simulink model "ballast_node"  (Simulink 7.8)
settings: Solver=FixedStepDiscrete  SolverMode=SingleTasking  StartTime=0.0  StopTime=10.0  FixedStep=0.01  RelTol=1e-3
InitFcn:
  | clear all
  | common
  | BallastBusses
undefined symbols (not defined in the file or in its folder): ANmax, BallastEcanInit, BallastNodeInit, Init_onlyOnce, Init_Reset, SendAndReceiveEcan, T_step
libraries: dsPICdrivers x11, simulink x6
settings Model: Creator=bwmairs  LastModifiedBy=Bryant
settings OptimizationCC: InlineParams=on  InlineInvariantSignals=on  InitFltsAndDblsToZero=on  EfficientFloat2IntCast=on
settings DebuggingCC: ReadBeforeWriteMsg=DisableAll  WriteAfterWriteMsg=DisableAll  WriteAfterReadMsg=DisableAll  UnderspecifiedInitializationDetection=Simplified  ParameterOverflowMsg=warning  FcnCallInpInsideContextMsg=Use local settings  UniqueDataStoreMsg=error
settings HardwareCC: ProdBitPerInt=16  ProdBitPerPointer=16  ProdIntDivRoundTo=Zero  ProdEndianess=LittleEndian  ProdWordSize=16  ProdHWDeviceType=16-bit Generic
settings ModelReferenceCC: ModelReferenceNumInstancesAllowed=Single
settings SFSimCC: SimParseCustomCode=off
settings RTWCC: SystemTargetFile=dspic.tlc  GenCodeOnly=on  MakeCommand=make_CreateMPLAB  TemplateMakefile=dspic_pic30_gcc.tmf  PostCodeGenCommand=dsPIC_Compile()  Description=Embedded Target for Microchip dsPIC (real-time)  ProcessScript=dspic_make_rtw_hook  RTWCompilerOptimization=On
settings RTWCC: CustomInclude=|
  | clib
  | ../Libs/C
settings RTWCC: CustomSource=|
  | clib/BallastNode.c
  | 
  | ../Libs/C/Node.c
  | ../Libs/C/Nmea2000.c
  | ../Libs/C/Nmea2000Encode.c
  | ../Libs/C/DEE.c
  | ../Libs/C/DEES_33F_24F.s
  | ../Libs/C/MessageScheduler.c
  | ../Libs/C/CanMessages.c
  | ../Libs/C/CircularBuffer.c
  | ../Libs/C/Ecan1.c
  | ../Libs/C/Parameters.c
  | ../Libs/C/ParametersHelper.c
  | ../Libs/C/DataStore.c
settings STFCustomTargetCC: TargetFunctionLibrary=C89/C90 (ANSI)  IncludeMdlTerminateFcn=off  SupportNonInlinedSFcns=off  SystemTargetFile=dspic.tlc
settings ERTTargetCC: TargetFunctionLibrary=C89/C90 (ANSI)  MultiwordLength=2048  ParMdlRefBuildCompliant=off  CompOptLevelCompliant=off  ConcurrentExecutionCompliant=off  IncludeMdlTerminateFcn=off  GeneratePreprocessorConditionals=Disable all  CombineOutputUpdateFcns=off  ERTFirstTimeCompliant=off  ERTCustomFileBanners=off  SupportContinuousTime=on  ModelStepFunctionPrototypeControlCompliant=off  CPPClassGenCompliant=off  ExtModeMexFile=ext_serial_win32_comm  InlinedParameterPlacement=NonHierarchical  ERTSrcFileBannerTemplate=dsPIC_code_template.cgt  ERTHdrFileBannerTemplate=dsPIC_code_template.cgt  ERTDataSrcFileTemplate=dsPIC_code_template.cgt  ERTDataHdrFileTemplate=dsPIC_code_template.cgt  ERTCustomFileTemplate=dsPIC_main.tlc  ConvertIfToSwitch=off  SuppressUnreachableDefaultCases=off
settings CustomProperty: DataType=string  Value=C:\PROGRA~1\MATLAB\R2011b\bin\win64\gmake

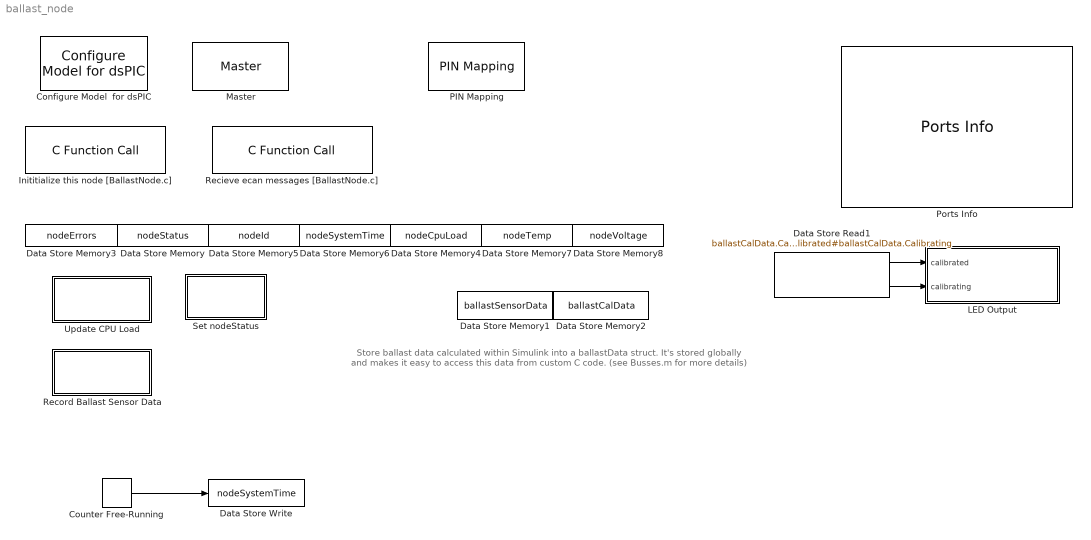
== system ballast_node ==
  note: Store ballast data calculated within Simulink into a ballastData struct.
      | It's stored globally and makes it easy to access this data from custom
      | C code. (see Busses.m for more details)
  Configure Model  for dsPIC : dsPICdrivers/Simulink Configuration/Configure Model  for dsPIC
  Counter Free-Running : simulink/Sources/Counter Free-Running  NumBits=32  tsamp=T_step
  Data Store Memory : DataStoreMemory  DataStoreName=nodeStatus  ReadBeforeWriteMsg=warning  WriteAfterWriteMsg=warning  WriteAfterReadMsg=warning  OutDataTypeStr=uint16
      settings: RTWStateStorageClass=ImportedExtern
  Data Store Memory1 : DataStoreMemory  DataStoreName=ballastSensorData  ReadBeforeWriteMsg=warning  WriteAfterWriteMsg=warning  WriteAfterReadMsg=warning  OutDataTypeStr=Bus: BallastVariables
      settings: RTWStateStorageClass=ImportedExtern
  Data Store Memory2 : DataStoreMemory  DataStoreName=ballastCalData  ReadBeforeWriteMsg=warning  WriteAfterWriteMsg=warning  WriteAfterReadMsg=warning  OutDataTypeStr=Bus: BallastCalData
      settings: RTWStateStorageClass=ImportedExtern
  Data Store Memory3 : DataStoreMemory  DataStoreName=nodeErrors  ReadBeforeWriteMsg=warning  WriteAfterWriteMsg=warning  WriteAfterReadMsg=warning  OutDataTypeStr=uint16
      settings: RTWStateStorageClass=ImportedExtern
  Data Store Memory4 : DataStoreMemory  DataStoreName=nodeCpuLoad  ReadBeforeWriteMsg=warning  WriteAfterWriteMsg=warning  WriteAfterReadMsg=warning  OutDataTypeStr=uint8
      settings: RTWStateStorageClass=ImportedExtern
  Data Store Memory5 : DataStoreMemory  DataStoreName=nodeId  ReadBeforeWriteMsg=warning  WriteAfterWriteMsg=warning  WriteAfterReadMsg=warning  OutDataTypeStr=uint8
      settings: RTWStateStorageClass=ImportedExtern
  Data Store Memory6 : DataStoreMemory  DataStoreName=nodeSystemTime  ReadBeforeWriteMsg=warning  WriteAfterWriteMsg=warning  WriteAfterReadMsg=warning  OutDataTypeStr=uint32
      settings: RTWStateStorageClass=ImportedExtern
  Data Store Memory7 : DataStoreMemory  DataStoreName=nodeTemp  ReadBeforeWriteMsg=warning  WriteAfterWriteMsg=warning  WriteAfterReadMsg=warning  OutDataTypeStr=int8
      settings: RTWStateStorageClass=ImportedExtern
  Data Store Memory8 : DataStoreMemory  DataStoreName=nodeVoltage  ReadBeforeWriteMsg=warning  WriteAfterWriteMsg=warning  WriteAfterReadMsg=warning  OutDataTypeStr=uint8
      settings: RTWStateStorageClass=ImportedExtern
  Data Store Read1 : DataStoreRead  DataStoreName=ballastCalData  SampleTime=T_step  DataStoreElements=ballastCalData.Calibrated#ballastCalData.Calibrating
  Data Store Write : DataStoreWrite  DataStoreName=nodeSystemTime
  Inititialize this node [BallastNode.c] : dsPICdrivers/OTHERS/C Function Call  Tag=dsPIC_dsPIC_CFunctionCall  FctUpdate=None  fctName=BallastEcanInit  INPUT_SIZE=1  INPUT1=--  INPUT2=--  INPUT3=--  OUTPUT_SIZE=-1  OUTPUT1=--  SampleTime=Inf  InputType=[]  OutputType=[]  FctDeclaration=extern void BallastEcanInit();  FctCall=BallastEcanInit();  OrderingInOutPopup=None  FctStart=Start Function (Call once and only once)  FctStart_Name=BallastNodeInit  FctStart_Declaration=inline extern void BallastNodeInit();  FctStart_Call=BallastNodeInit();  FctInit=None  FctInit_Name=BallastEcanInit  FctInit_Declaration=inline extern void BallastEcanInit();  FctInit_Call=BallastEcanInit();  PinDigitalInput=[]  PinDigitalOutput=[]  AnalogueInput=[]
  LED Output : Subsystem
  Master : dsPICdrivers/Master  Tag=dsPIC_MASTER  Priority=1  TimeStepType=Timer1  picType=33fj128MC802  fcy=40008571.4286  Quartz_33f=8e6  PLLActive_33f=on  fcyDesired_33f=40000000  tmr1="[8  50010  -0.00057131]"  tmr1Info="Time Step : 0.01  ;   Error : -0.00057131%  PR1=50010"  tmr2345="[0  0  0  0]"  tmr2345cfg=[-1 -1 -1 -1]  IOautoConf=on  typePort="[ 9   8   0   0  10   0   0   0   0   0   0   0   0   0   0   0   0   9   8   8  22   0   0  23   0   0   0   0  23   0   0   0   0   0   0   0   0   0   0   0   0   0   0   0   0   0   0   0   0   0   0   0   0   0   0   0   0   0   0   0   0   0   0   0   0   0   0   0   0   0   0   0   0   0   0   0   0   0   0   0   0   0   0   0   0   0   0   0   0   0   0   0   0   0   0   0   0   0   0   0   0   0   0   0   0   0   0   0   0   0   0   0 ]"  TRIS="[ 65519  61311  65535  65535  65535  65535  65535 ]"  ADPCFG=9  MasterBusyPort=None  MasterOverloadPort=None  FOSC=Internal Fast RC 7.37Mhz  ClockSwitchMonitor=Both disabled  TempProtection_33f=TEMP_ON  FPBOR=<empty>  PWRT=disable  MCLR=<empty>  ICD=ICS_PGD3  JTAGEN=JTAGEN_OFF  PowerSave=off  OverrideFcy=off  NewFcy=1e6  PR2345="[65535  65535  65535  65535]"
  PIN Mapping : dsPICdrivers/Peripheral MAPPING/PIN Mapping  Tag=dsPIC_PIN_Mapping  in_INT1=Not tied (VSS)  in_INT2=Not tied (VSS)  in_T2CK=Not tied (VSS)  in_T3CK=Not tied (VSS)  in_T4CK=Not tied (VSS)  in_T5CK=Not tied (VSS)  in_IC1=Not tied (VSS)  in_IC2=Not tied (VSS)  in_IC7=Not tied (VSS)  in_IC8=Not tied (VSS)  out_OC1=tied to RP12  out_OC2=Not changed  out_OC3=Not changed  out_OC4=Not changed  in_OCFA=Not tied (VSS)  in_FLTA1=Not tied (VSS)  in_FLTA2=Not tied (VSS)  in_QEA1=Not tied (VSS)  in_QEB1=Not tied (VSS)  in_INDX1=Not tied (VSS)  out_UPDN1=Not changed  out_UPDN2=Not changed  in_QEA2=Not tied (VSS)  in_QEB2=Not tied (VSS)  in_INDX2=Not tied (VSS)  in_U1RX=Not tied (VSS)  out_U1TX=Not changed  in_U1CTS=Not tied (VSS)  out_U1RTS=Not changed  in_U2RX=Not tied (VSS)  out_U2TX=Not changed  in_U2CTS=Not tied (VSS)  out_U2RTS=Not changed  in_SDI1=Not tied (VSS)  out_SDO1=Not changed  in_SCK1=Not tied (VSS)  out_SCK1OUT=Not changed  in_SS1=Not tied (VSS)  out_SS1OUT=Not changed  in_SDI2=Not tied (VSS)  out_SDO2=Not changed  in_SCK2=Not tied (VSS)  out_SCK2OUT=Not changed  in_SS2=Not tied (VSS)  out_SS2OUT=Not changed  in_C1RX=tied to RP4  out_C1TX=tied to RP7  out_C1OUT=Not changed  out_C2OUT=Not changed
  Ports Info : dsPICdrivers/Ports Info  Tag=dsPIC_PortInfo
  Recieve ecan messages [BallastNode.c] : dsPICdrivers/OTHERS/C Function Call  Tag=dsPIC_dsPIC_CFunctionCall  FctUpdate=Output Function  fctName=SendAndReceiveEcan  INPUT_SIZE=1  INPUT1=--  INPUT2=--  INPUT3=--  OUTPUT_SIZE=1  OUTPUT1=--  SampleTime=.01  InputType=[ ]  OutputType=[ ]  FctDeclaration=extern void SendAndReceiveEcan();  FctCall=SendAndReceiveEcan();  OrderingInOutPopup=None  FctStart=None  FctStart_Name=Init_onlyOnce  FctStart_Declaration=inline extern void Init_onlyOnce();  FctStart_Call=Init_onlyOnce();  FctInit=None  FctInit_Name=Init_Reset  FctInit_Declaration=inline extern void Init_Reset();  FctInit_Call=Init_Reset();  PinDigitalInput=[]  PinDigitalOutput=[]  AnalogueInput=[]
  Record Ballast Sensor Data : Subsystem
  Set nodeStatus : Subsystem
  Update CPU Load : Subsystem
      mask Display: disp('');
  wires:
  Data Store Read1/1 -> LED Output/1(calibrated)
  Data Store Read1/2 -> LED Output/2(calibrating)
  Counter Free-Running/1 -> Data Store Write/1

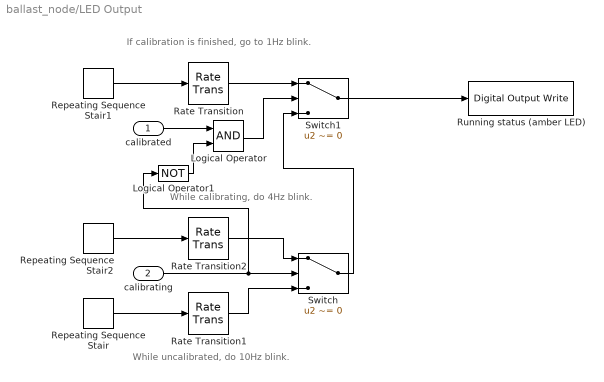
== system ballast_node/LED Output ==
  note: If calibration is finished, go to 1Hz blink.
  note: While calibrating, do 4Hz blink.
  note: While uncalibrated, do 10Hz blink.
  calibrated : Inport
  calibrating : Inport  Port=2
  Logical Operator : Logic  AllPortsSameDT=off  OutDataTypeStr=boolean
  Logical Operator1 : Logic  Operator=NOT  AllPortsSameDT=off  OutDataTypeStr=boolean
  Rate Transition : RateTransition
  Rate Transition1 : RateTransition
  Rate Transition2 : RateTransition
  Repeating Sequence Stair : simulink/Sources/Repeating Sequence Stair  OutValues=[1 0]  tsamp=.1  OutMin=[]  OutMax=[]  OutDataTypeStr=fixdt('boolean')  OutputDataTypeScalingMode=Specify via dialog  OutDataType=fixdt('boolean')  ConRadixGroup=Best Precision: Vector-wise  OutScaling=[]
  Repeating Sequence Stair1 : simulink/Sources/Repeating Sequence Stair  OutValues=[1 0]  tsamp=1  OutMin=[]  OutMax=[]  OutDataTypeStr=fixdt('boolean')  OutputDataTypeScalingMode=Specify via dialog  OutDataType=fixdt('boolean')  ConRadixGroup=Best Precision: Vector-wise  OutScaling=[]
  Repeating Sequence Stair2 : simulink/Sources/Repeating Sequence Stair  OutValues=[1 0]  tsamp=.25  OutMin=[]  OutMax=[]  OutDataTypeStr=fixdt('boolean')  OutputDataTypeScalingMode=Specify via dialog  OutDataType=fixdt('boolean')  ConRadixGroup=Best Precision: Vector-wise  OutScaling=[]
  Running status (amber LED) : dsPICdrivers/Digital I//O/Digital Output Write  Tag=dsPIC_Digital_Output  Priority=5  PORT=A  Pin=[4]  Simultaneous=off  OrderingInOutPopup=None
  Switch : Switch  Criteria=u2 ~= 0
  Switch1 : Switch  Criteria=u2 ~= 0
  wires:
  Repeating Sequence Stair/1 -> Rate Transition1/1
  Rate Transition1/1 -> Switch/3
  calibrating/1 -> Switch/2, Logical Operator1/1
  Repeating Sequence Stair1/1 -> Rate Transition/1
  Rate Transition/1 -> Switch1/1
  Repeating Sequence Stair2/1 -> Rate Transition2/1
  Rate Transition2/1 -> Switch/1
  Switch1/1 -> Running status (amber LED)/1
  Switch/1 -> Switch1/3
  calibrated/1 -> Logical Operator/1
  Logical Operator/1 -> Switch1/2
  Logical Operator1/1 -> Logical Operator/2

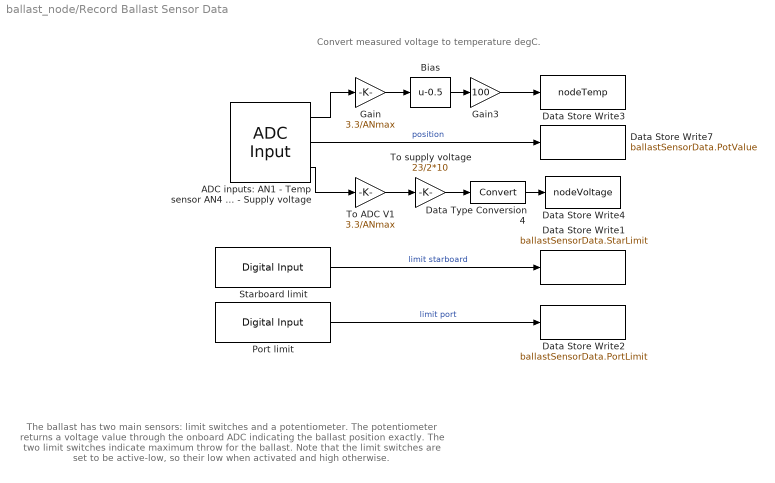
== system ballast_node/Record Ballast Sensor Data ==
  note: The ballast has two main sensors: limit switches and a potentiometer. The
      | potentiometer returns a voltage value through the onboard ADC indicating
      | the ballast position exactly. The two limit switches indicate maximum throw
      | for the ballast.
      |
      | Note that the limit switches are set to be active-low, so their low when activated
      | and high otherwise.
  note: Convert measured voltage to temperature degC.
  ADC inputs: AN1 - Temp sensor AN4 - Ballast pot AN5 - Supply voltage : dsPICdrivers/Peripheral I//O/ADC Input  Tag=dsPIC_ADC  Priority=5  ADC_TYPE=12 bits  ADC_MODE=Continuous sampling & get last channel value  NbrSampleStep=1  VoltRefpopup="AVdd  -  AVss"  OutFormatBitspopup=0000 dddd dddd dddd : Integer  InterruptPriority=6  ANCHANNELS=[4 5 1]  MaxName=ANmax = 4095  Rin=0  ADCS=53  SAMC=1  Temperature=25  DMAChannel=1  SampleTime=T_step  Status="OK  |  Tsmp=6.749e-007 |  T/Channel=1.012e-005 |  Tall=3.037e-005"  SSRC=auto convert
  Bias : Bias  Bias=-0.5
  Data Store Write1 : DataStoreWrite  DataStoreName=ballastSensorData  DataStoreElements=ballastSensorData.StarLimit
  Data Store Write2 : DataStoreWrite  DataStoreName=ballastSensorData  DataStoreElements=ballastSensorData.PortLimit
  Data Store Write3 : DataStoreWrite  DataStoreName=nodeTemp
  Data Store Write4 : DataStoreWrite  DataStoreName=nodeVoltage
  Data Store Write7 : DataStoreWrite  DataStoreName=ballastSensorData  DataStoreElements=ballastSensorData.PotValue
  Data Type Conversion4 : DataTypeConversion  RndMeth=Simplest
  Gain : Gain  Gain=3.3/ANmax  ParamDataTypeStr=single  OutDataTypeStr=single  RndMeth=Simplest
  Gain3 : Gain  Gain=100  ParamDataTypeStr=single  OutDataTypeStr=int8  RndMeth=Simplest
  Port limit : dsPICdrivers/Digital I//O/Digital Input  Tag=dsPIC_Digital_Input  PORT=A  Pin=[0]  SampleTime=T_step  OrderingInOutPopup=None
  Starboard limit : dsPICdrivers/Digital I//O/Digital Input  Tag=dsPIC_Digital_Input  PORT=B  Pin=[1]  SampleTime=T_step  OrderingInOutPopup=None
  To ADC V1 : Gain  Gain=3.3/ANmax
  To supply voltage : Gain  Gain=23/2*10  RndMeth=Simplest
  wires:
  Port limit/1 -> Data Store Write2/1  "limit port"
  Starboard limit/1 -> Data Store Write1/1  "limit starboard"
  ADC inputs: AN1 - Temp sensor AN4 - Ballast pot AN5 - Supply voltage/1 -> Gain/1
  Gain/1 -> Bias/1
  Bias/1 -> Gain3/1
  Gain3/1 -> Data Store Write3/1
  To ADC V1/1 -> To supply voltage/1
  ADC inputs: AN1 - Temp sensor AN4 - Ballast pot AN5 - Supply voltage/3 -> To ADC V1/1
  To supply voltage/1 -> Data Type Conversion4/1
  Data Type Conversion4/1 -> Data Store Write4/1
  ADC inputs: AN1 - Temp sensor AN4 - Ballast pot AN5 - Supply voltage/2 -> Data Store Write7/1  "position"

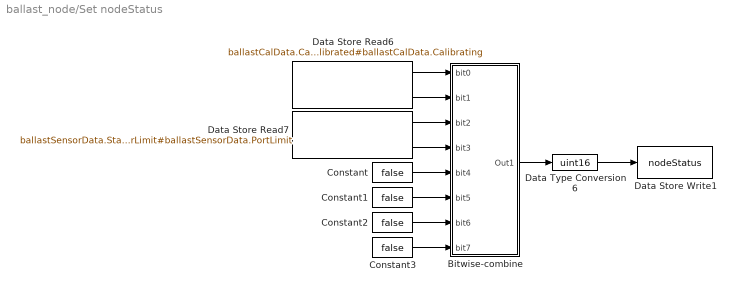
== system ballast_node/Set nodeStatus ==
  Bitwise-combine : Subsystem
  Constant{,1..3} (4 alike) : Constant  Value=false  OutDataTypeStr=boolean
  Data Store Read6 : DataStoreRead  DataStoreName=ballastCalData  SampleTime=T_step  DataStoreElements=ballastCalData.Calibrated#ballastCalData.Calibrating
  Data Store Read7 : DataStoreRead  DataStoreName=ballastSensorData  SampleTime=T_step  DataStoreElements=ballastSensorData.StarLimit#ballastSensorData.PortLimit
  Data Store Write1 : DataStoreWrite  DataStoreName=nodeStatus
  Data Type Conversion6 : DataTypeConversion  OutDataTypeStr=uint16
  wires:
  Constant/1 -> Bitwise-combine/5(bit4)
  Constant1/1 -> Bitwise-combine/6(bit5)
  Constant2/1 -> Bitwise-combine/7(bit6)
  Constant3/1 -> Bitwise-combine/8(bit7)
  Data Store Read6/1 -> Bitwise-combine/1(bit0)
  Data Store Read6/2 -> Bitwise-combine/2(bit1)
  Data Store Read7/1 -> Bitwise-combine/3(bit2)
  Data Store Read7/2 -> Bitwise-combine/4(bit3)
  Bitwise-combine/1(Out1) -> Data Type Conversion6/1
  Data Type Conversion6/1 -> Data Store Write1/1

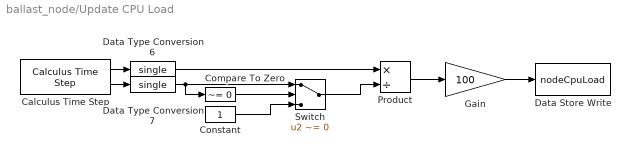
== system ballast_node/Update CPU Load ==
  Calculus Time Step : dsPICdrivers/OTHERS/Calculus Time Step  Tag=dsPIC_CalculusTimeStep  SampleTime=1  PR1chk=on
  Compare To Zero : simulink/Logic and Bit Operations/Compare To Zero  relop=~=  OutDataTypeStr=uint8
  Constant : Constant
  Data Store Write : DataStoreWrite  DataStoreName=nodeCpuLoad
  Data Type Conversion6 : DataTypeConversion  OutDataTypeStr=single
  Data Type Conversion7 : DataTypeConversion  OutDataTypeStr=single
  Gain : Gain  Gain=100  OutDataTypeStr=uint8
  Product : Product  Inputs=*/  RndMeth=Zero
  Switch : Switch  Criteria=u2 ~= 0
  wires:
  Constant/1 -> Switch/3
  Compare To Zero/1 -> Switch/2
  Switch/1 -> Product/2
  Data Type Conversion7/1 -> Compare To Zero/1, Switch/1
  Data Type Conversion6/1 -> Product/1
  Gain/1 -> Data Store Write/1
  Product/1 -> Gain/1
  Calculus Time Step/2 -> Data Type Conversion7/1
  Calculus Time Step/1 -> Data Type Conversion6/1

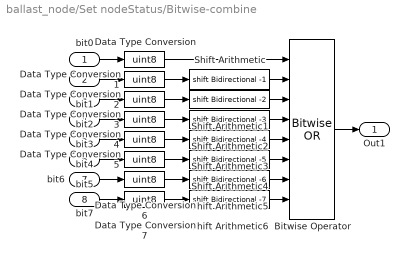
== system ballast_node/Set nodeStatus/Bitwise-combine ==
  bit0 : Inport
  bit1 : Inport  Port=2
  bit2 : Inport  Port=3
  bit3 : Inport  Port=4
  bit4 : Inport  Port=5
  bit5 : Inport  Port=6
  bit6 : Inport  Port=7
  bit7 : Inport  Port=8
  Bitwise Operator : simulink/Logic and Bit Operations/Bitwise Operator  logicop=OR  UseBitMask=off  NumInputPorts=8  BitMask=bin2dec('11011001')  BitMaskRealWorld=Stored Integer
  Data Type Conversion{,1..7} (8 alike) : DataTypeConversion  OutDataTypeStr=uint8
  Shift Arithmetic : ArithShift  BitShiftNumber=-1
  Shift Arithmetic1 : ArithShift  BitShiftNumber=-2
  Shift Arithmetic2 : ArithShift  BitShiftNumber=-3
  Shift Arithmetic3 : ArithShift  BitShiftNumber=-4
  Shift Arithmetic4 : ArithShift  BitShiftNumber=-5
  Shift Arithmetic5 : ArithShift  BitShiftNumber=-6
  Shift Arithmetic6 : ArithShift  BitShiftNumber=-7
  Out1 : Outport
  wires:
  Shift Arithmetic/1 -> Bitwise Operator/2
  Shift Arithmetic1/1 -> Bitwise Operator/3
  Shift Arithmetic2/1 -> Bitwise Operator/4
  Data Type Conversion/1 -> Bitwise Operator/1
  Data Type Conversion1/1 -> Shift Arithmetic/1
  Data Type Conversion2/1 -> Shift Arithmetic1/1
  Data Type Conversion3/1 -> Shift Arithmetic2/1
  Data Type Conversion4/1 -> Shift Arithmetic3/1
  Shift Arithmetic3/1 -> Bitwise Operator/5
  Data Type Conversion5/1 -> Shift Arithmetic4/1
  Data Type Conversion6/1 -> Shift Arithmetic5/1
  Shift Arithmetic4/1 -> Bitwise Operator/6
  Shift Arithmetic5/1 -> Bitwise Operator/7
  Data Type Conversion7/1 -> Shift Arithmetic6/1
  Shift Arithmetic6/1 -> Bitwise Operator/8
  bit0/1 -> Data Type Conversion/1
  bit1/1 -> Data Type Conversion1/1
  bit2/1 -> Data Type Conversion2/1
  bit3/1 -> Data Type Conversion3/1
  Bitwise Operator/1 -> Out1/1
  bit4/1 -> Data Type Conversion4/1
  bit5/1 -> Data Type Conversion5/1
  bit6/1 -> Data Type Conversion6/1
  bit7/1 -> Data Type Conversion7/1
